simulink model "TRAS_PID_Cross"  (R2016a)
settings: Solver=ode5  SolverMode=SingleTasking  StartTime=0.0  StopTime=90  FixedStep=0.01  RelTol=1e-3  AbsTol=1e-6
settings Model: SimulationMode=external  ExtModeTrigDuration=12000  ExtModeTrigLevel=0.400000  Creator=jims  LastModifiedBy=inteco
settings DataIOCC: ExternalInput=[]  InitialState=[]  MaxDataPoints=5000  SaveFormat=Array  SignalLoggingSaveFormat=ModelDataLogs  SaveOutput=off  SaveTime=off  SignalLoggingName=sigsOut
settings OptimizationCC: BooleanDataType=off  ExpressionDepthLimit=2147483647  InitFltsAndDblsToZero=on
settings DebuggingCC: SaveWithParameterizedLinksMsg=none  UnderspecifiedInitializationDetection=Classic  MergeDetectMultiDrivingBlocksExec=none  SignalResolutionControl=TryResolveAllWithWarning  MultiTaskDSMMsg=warning  MultiTaskCondExecSysMsg=none  IntegerOverflowMsg=none  FcnCallInpInsideContextMsg=UseLocalSettings  StateNameClashWarn=warning  IntegerSaturationMsg=none
settings HardwareCC: ProdBitPerPointer=32  ProdLargestAtomicFloat=None  ProdIntDivRoundTo=Undefined  ProdEndianess=Unspecified  ProdWordSize=32  ProdHWDeviceType=32-bit Generic
settings ModelReferenceCC: PropagateSignalLabelsOutOfModel=off
settings RTWCC: SystemTargetFile=rtcon_tras_usb2.tlc  TemplateMakefile=rtcon_tras_vc_usb2_x64.tmf  Description=TRAS RTDAC/USB2 (Visual C/C++)
settings STFCustomTargetCC: ModelReferenceCompliant=off  GeneratePreprocessorConditionals=Disable all  CombineOutputUpdateFcns=on  MatFileLogging=on  CPPClassGenCompliant=on  GRTInterface=off  SystemTargetFile=rtcon_tras_usb2.tlc
settings GRTTargetCC: ModelReferenceCompliant=off  ParMdlRefBuildCompliant=off  CompOptLevelCompliant=off  ConcurrentExecutionCompliant=off  UseToolchainInfoCompliant=off  ExtMode=on  ExtModeMexFile=rtcon_ext_comm
settings ConfigComp: CovModelRefEnable=Off  CovSFcnEnable=off

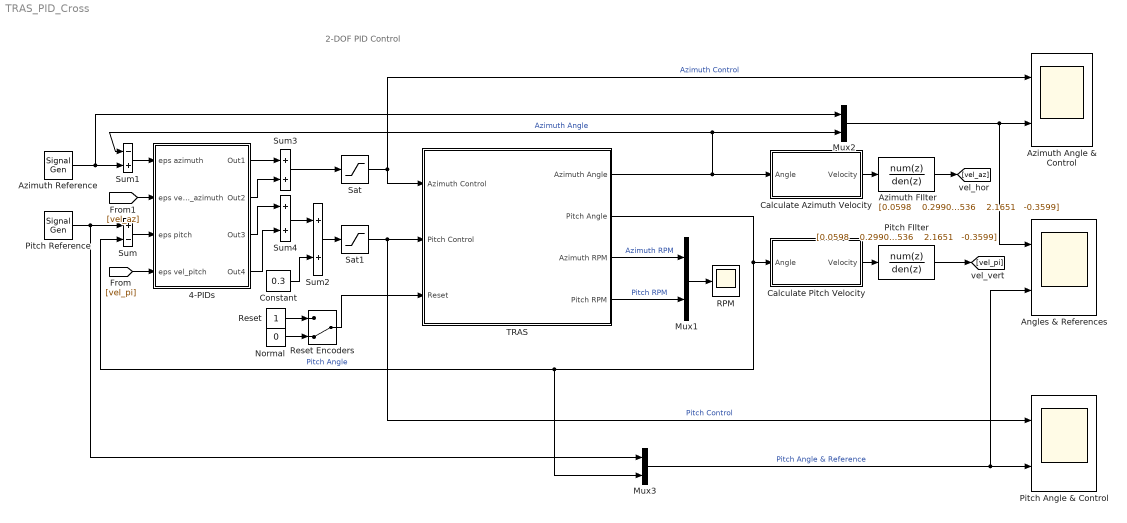
== system TRAS_PID_Cross ==
  note: 2-DOF PID Control
  4-PIDs : Subsystem  mask(4 PID controllers){phh=[1.9758/1.5 0.115 1.4008], pvh=[0 0 0.3], phv=[0 0 0.223], pvv=[0.0339 0.3532 0.7918]}
      mask prompts: phh "[Kphh Kihh Kdhh]"; pvh "[Kpvh Kivh Kdvh]"; phv "[Kphv Kihv Kdhv]"; pvv "[Kpvv Kivv Kdvv]"
      mask help: Parameters for cross-coupled PID controllers
      mask init:
      | Kphh = phh(1); Kihh = phh(2); Kdhh = phh(3);
      | Kpvh = pvh(1); Kivh = pvh(2); Kdvh = pvh(3);
      | Kphv = phv(1); Kihv = phv(2); Kdhv = phv(3);
      | Kpvv = pvv(1); Kivv = pvv(2); Kdvv = pvv(3);
      mask Help: Parameters for cross-coupled PID controllers
  Angles & References : Scope  NumInputPorts=2
  Azimuth Angle & Control : Scope  NumInputPorts=2
  Azimuth Reference : SignalGenerator  WaveForm=square  Amplitude=.4  Frequency=.02
  Azimuth FIlter : DiscreteTransferFcn  Numerator="[0.0598    0.2990    0.5980    0.5980    0.2990    0.0598] * 1e-3"  Denominator="[1.0000   -3.9845    6.4349   -5.2536    2.1651   -0.3599]"  SampleTime=0.01
  Calculate Azimuth Velocity : Subsystem
      mask Display: disp( 'rad-to-rad/s' )
  Calculate Pitch Velocity : Subsystem
      mask Display: disp( 'rad-to-rad/s' )
  Constant : Constant  Value=0.3
  Mux1 : Mux  Inputs=2
  Mux2 : Mux  Inputs=2
  Mux3 : Mux  Inputs=2
  Normal : Constant  Value=0
  Pitch Angle & Control : Scope  NumInputPorts=2
  Pitch Reference : SignalGenerator  Amplitude=.25  Frequency=1/60
  Pitch FIlter : DiscreteTransferFcn  Numerator="[0.0598    0.2990    0.5980    0.5980    0.2990    0.0598] * 1e-3"  Denominator="[1.0000   -3.9845    6.4349   -5.2536    2.1651   -0.3599]"  SampleTime=0.01
  RPM : Scope
  Reset : Constant
  Reset Encoders : ManualSwitch  CurrentSetting=0
  Sat : Saturate
  Sat1 : Saturate  UpperLimit=1  LowerLimit=0
  Sum : Sum  Inputs=+-  SaturateOnIntegerOverflow=on
  Sum1 : Sum  Inputs=-+  SaturateOnIntegerOverflow=on
  Sum2 : Sum  SaturateOnIntegerOverflow=on
  Sum3 : Sum  SaturateOnIntegerOverflow=on
  Sum4 : Sum  SaturateOnIntegerOverflow=on
  TRAS : Subsystem
      mask Display: image(imread('Tras.JPG'))
  wires:
  TRAS/1(Azimuth Angle) -> Mux2/2, Sum1/1, Calculate Azimuth Velocity/1(Angle)  "Azimuth Angle"
  TRAS/4(Pitch RPM) -> Mux1/2  "Pitch RPM"
  Normal/1 -> Reset Encoders/2
  Reset/1 -> Reset Encoders/1
  Reset Encoders/1 -> TRAS/3(Reset)
  Mux2/1 -> Angles & References/1, Azimuth Angle & Control/2
  Sum2/1 -> Sat1/1
  Sat1/1 -> Pitch Angle & Control/1, TRAS/2(Pitch Control)  "Pitch Control"
  Azimuth Reference/1 -> Sum1/2, Mux2/1
  Pitch Reference/1 -> Sum/1, Mux3/1
  Sat/1 -> Azimuth Angle & Control/1, TRAS/1(Azimuth Control)  "Azimuth Control"
  Constant/1 -> Sum2/2
  Sum3/1 -> Sat/1
  Sum4/1 -> Sum2/1
  Mux1/1 -> RPM/1
  TRAS/2(Pitch Angle) -> Sum/2, Mux3/2, Calculate Pitch Velocity/1(Angle)  "Pitch Angle"
  Mux3/1 -> Angles & References/2, Pitch Angle & Control/2  "Pitch Angle & Reference"
  Calculate Azimuth Velocity/1(Velocity) -> Azimuth FIlter/1
  Calculate Pitch Velocity/1(Velocity) -> Pitch FIlter/1
  Sum1/1 -> 4-PIDs/1(eps azimuth)
  Sum/1 -> 4-PIDs/3(eps pitch)
  Azimuth FIlter/1 -> [vel_az]
  Pitch FIlter/1 -> [vel_pi]
  4-PIDs/1(Out1) -> Sum3/1
  4-PIDs/2(Out2) -> Sum3/2
  4-PIDs/3(Out3) -> Sum4/1
  4-PIDs/4(Out4) -> Sum4/2
  [vel_az] -> 4-PIDs/2(eps vel_azimuth)
  [vel_pi] -> 4-PIDs/4(eps vel_pitch)
  TRAS/3(Azimuth RPM) -> Mux1/1  "Azimuth RPM"

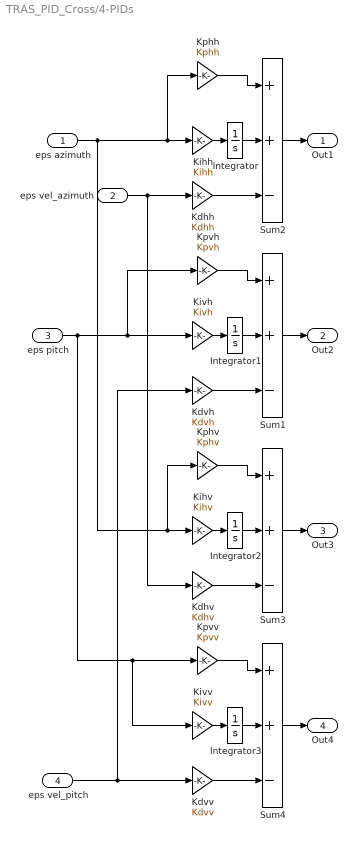
== system TRAS_PID_Cross/4-PIDs ==
  eps azimuth : Inport
  eps vel_azimuth : Inport  Port=2
  eps pitch : Inport  Port=3
  eps vel_pitch : Inport  Port=4
  Integrator : Integrator  LimitOutput=on  UpperSaturationLimit=0.5  LowerSaturationLimit=-0.5
  Integrator1 : Integrator  LimitOutput=on
  Integrator2 : Integrator
  Integrator3 : Integrator  LimitOutput=on  UpperSaturationLimit=0.25  LowerSaturationLimit=-0.25
  Kdhh : Gain  Gain=Kdhh  SaturateOnIntegerOverflow=on  OutDataTypeStr=Inherit: Same as input  ParamDataTypeStr=Inherit: Same as input
  Kdhv : Gain  Gain=Kdhv  SaturateOnIntegerOverflow=on  OutDataTypeStr=Inherit: Same as input  ParamDataTypeStr=Inherit: Same as input
  Kdvh : Gain  Gain=Kdvh  SaturateOnIntegerOverflow=on  OutDataTypeStr=Inherit: Same as input  ParamDataTypeStr=Inherit: Same as input
  Kdvv : Gain  Gain=Kdvv  SaturateOnIntegerOverflow=on  OutDataTypeStr=Inherit: Same as input  ParamDataTypeStr=Inherit: Same as input
  Kihh : Gain  Gain=Kihh  SaturateOnIntegerOverflow=on  OutDataTypeStr=Inherit: Same as input  ParamDataTypeStr=Inherit: Same as input
  Kihv : Gain  Gain=Kihv  SaturateOnIntegerOverflow=on  OutDataTypeStr=Inherit: Same as input  ParamDataTypeStr=Inherit: Same as input
  Kivh : Gain  Gain=Kivh  SaturateOnIntegerOverflow=on  OutDataTypeStr=Inherit: Same as input  ParamDataTypeStr=Inherit: Same as input
  Kivv : Gain  Gain=Kivv  SaturateOnIntegerOverflow=on  OutDataTypeStr=Inherit: Same as input  ParamDataTypeStr=Inherit: Same as input
  Kphh : Gain  Gain=Kphh  SaturateOnIntegerOverflow=on  OutDataTypeStr=Inherit: Same as input  ParamDataTypeStr=Inherit: Same as input
  Kphv : Gain  Gain=Kphv  SaturateOnIntegerOverflow=on  OutDataTypeStr=Inherit: Same as input  ParamDataTypeStr=Inherit: Same as input
  Kpvh : Gain  Gain=Kpvh  SaturateOnIntegerOverflow=on  OutDataTypeStr=Inherit: Same as input  ParamDataTypeStr=Inherit: Same as input
  Kpvv : Gain  Gain=Kpvv  SaturateOnIntegerOverflow=on  OutDataTypeStr=Inherit: Same as input  ParamDataTypeStr=Inherit: Same as input
  Sum{1..4} (4 alike) : Sum  Inputs=++-  SaturateOnIntegerOverflow=on  InputSameDT=on  OutDataTypeStr=Inherit: Same as first input
  Out1 : Outport
  Out2 : Outport  Port=2
  Out3 : Outport  Port=3
  Out4 : Outport  Port=4
  wires:
  Sum4/1 -> Out4/1
  Sum3/1 -> Out3/1
  Sum1/1 -> Out2/1
  Sum2/1 -> Out1/1
  Kdvv/1 -> Sum4/3
  Kivv/1 -> Integrator3/1
  Integrator3/1 -> Sum4/2
  Kpvv/1 -> Sum4/1
  Kdhv/1 -> Sum3/3
  Kihv/1 -> Integrator2/1
  Integrator2/1 -> Sum3/2
  Kphv/1 -> Sum3/1
  Kdvh/1 -> Sum1/3
  Kivh/1 -> Integrator1/1
  Integrator1/1 -> Sum1/2
  Kpvh/1 -> Sum1/1
  Kdhh/1 -> Sum2/3
  Kihh/1 -> Integrator/1
  Integrator/1 -> Sum2/2
  Kphh/1 -> Sum2/1
  eps azimuth/1 -> Kihv/1, Kphv/1, Kihh/1, Kphh/1
  eps vel_azimuth/1 -> Kdhv/1, Kdhh/1
  eps pitch/1 -> Kivh/1, Kpvh/1, Kpvv/1, Kivv/1
  eps vel_pitch/1 -> Kdvv/1, Kdvh/1

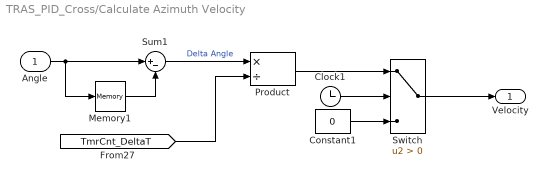
== system TRAS_PID_Cross/Calculate Azimuth Velocity ==
  Angle : Inport
  Clock1 : Clock
  Constant1 : Constant  Value=0
  Memory1 : Memory
  Product : Product  Inputs=*/  SaturateOnIntegerOverflow=on  InputSameDT=on  OutDataTypeStr=Inherit: Same as first input
  Sum1 : Sum  Inputs=|+-  SaturateOnIntegerOverflow=on  InputSameDT=on  OutDataTypeStr=Inherit: Same as first input
  Switch : Switch  Criteria=u2 > Threshold  SaturateOnIntegerOverflow=on  InputSameDT=on
  Velocity : Outport
  wires:
  [TmrCnt_DeltaT] -> Product/2
  Memory1/1 -> Sum1/2
  Angle/1 -> Sum1/1, Memory1/1
  Sum1/1 -> Product/1  "Delta Angle"
  Product/1 -> Switch/1
  Clock1/1 -> Switch/2
  Constant1/1 -> Switch/3
  Switch/1 -> Velocity/1

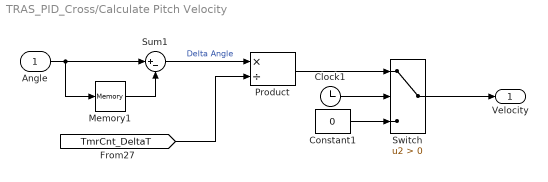
== system TRAS_PID_Cross/Calculate Pitch Velocity ==
  Angle : Inport
  Clock1 : Clock
  Constant1 : Constant  Value=0
  Memory1 : Memory
  Product : Product  Inputs=*/  SaturateOnIntegerOverflow=on  InputSameDT=on  OutDataTypeStr=Inherit: Same as first input
  Sum1 : Sum  Inputs=|+-  SaturateOnIntegerOverflow=on  InputSameDT=on  OutDataTypeStr=Inherit: Same as first input
  Switch : Switch  Criteria=u2 > Threshold  SaturateOnIntegerOverflow=on  InputSameDT=on
  Velocity : Outport
  wires:
  Switch/1 -> Velocity/1
  Constant1/1 -> Switch/3
  Clock1/1 -> Switch/2
  Product/1 -> Switch/1
  Sum1/1 -> Product/1  "Delta Angle"
  Angle/1 -> Memory1/1, Sum1/1
  Memory1/1 -> Sum1/2
  [TmrCnt_DeltaT] -> Product/2

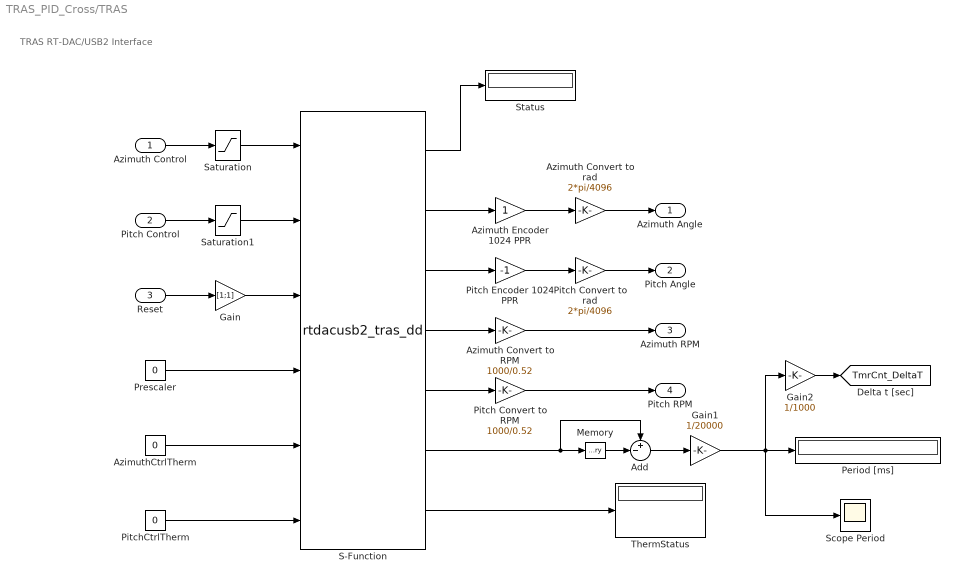
== system TRAS_PID_Cross/TRAS ==
  note: TRAS RT-DAC/USB2
      | Interface
  Azimuth Control : Inport
  Pitch Control : Inport  Port=2
  Reset : Inport  Port=3
  Add : Sum  Inputs=+-|
  Azimuth Convert to RPM : Gain  Gain=1000/0.52  SaturateOnIntegerOverflow=on  OutDataTypeStr=Inherit: Same as input  ParamDataTypeStr=Inherit: Same as input
  Azimuth Convert to rad : Gain  Gain=2*pi/4096  SaturateOnIntegerOverflow=on  OutDataTypeStr=Inherit: Same as input  ParamDataTypeStr=Inherit: Same as input
  Azimuth Encoder 1024 PPR : Gain  SaturateOnIntegerOverflow=on  OutDataTypeStr=Inherit: Same as input  ParamDataTypeStr=Inherit: Same as input
  AzimuthCtrlTherm : Constant  Value=0
  Gain : Gain  Gain=[1;1]
  Gain1 : Gain  Gain=1/20000
  Gain2 : Gain  Gain=1/1000
  Memory : Memory
  Period [ms] : Display
  Pitch Convert to RPM : Gain  Gain=1000/0.52  SaturateOnIntegerOverflow=on  OutDataTypeStr=Inherit: Same as input  ParamDataTypeStr=Inherit: Same as input
  Pitch Convert to rad : Gain  Gain=2*pi/4096  SaturateOnIntegerOverflow=on  OutDataTypeStr=Inherit: Same as input  ParamDataTypeStr=Inherit: Same as input
  Pitch Encoder 1024 PPR : Gain  Gain=-1  SaturateOnIntegerOverflow=on  OutDataTypeStr=Inherit: Same as input  ParamDataTypeStr=Inherit: Same as input
  PitchCtrlTherm : Constant  Value=0
  Prescaler : Constant  Value=0
  S-Function : S-Function  FunctionName=rtdacusb2_tras_dd  Parameters=1, 0.01  SFunctionDeploymentMode=off  EnableBusSupport=off
  Saturation : Saturate  UpperLimit=1  LowerLimit=-1
  Saturation1 : Saturate  UpperLimit=1  LowerLimit=-1
  Scope Period : Scope
  Status : Display
  ThermStatus : Display
  Azimuth Angle : Outport
  Pitch Angle : Outport  Port=2
  Azimuth RPM : Outport  Port=3
  Pitch RPM : Outport  Port=4
  tag scope: TmrCnt_DeltaT=global
  wires:
  Gain2/1 -> [TmrCnt_DeltaT]
  Gain1/1 -> Gain2/1, Period [ms]/1, Scope Period/1
  S-Function/6 -> Add/1, Memory/1
  Add/1 -> Gain1/1
  Memory/1 -> Add/2
  S-Function/7 -> ThermStatus/1
  Pitch Convert to RPM/1 -> Pitch RPM/1
  Azimuth Convert to RPM/1 -> Azimuth RPM/1
  S-Function/5 -> Pitch Convert to RPM/1
  S-Function/4 -> Azimuth Convert to RPM/1
  Pitch Convert to rad/1 -> Pitch Angle/1
  S-Function/3 -> Pitch Encoder 1024 PPR/1
  Pitch Encoder 1024 PPR/1 -> Pitch Convert to rad/1
  Azimuth Convert to rad/1 -> Azimuth Angle/1
  S-Function/2 -> Azimuth Encoder 1024 PPR/1
  Azimuth Encoder 1024 PPR/1 -> Azimuth Convert to rad/1
  S-Function/1 -> Status/1
  Gain/1 -> S-Function/3
  Saturation1/1 -> S-Function/2
  Saturation/1 -> S-Function/1
  PitchCtrlTherm/1 -> S-Function/6
  AzimuthCtrlTherm/1 -> S-Function/5
  Prescaler/1 -> S-Function/4
  Reset/1 -> Gain/1
  Pitch Control/1 -> Saturation1/1
  Azimuth Control/1 -> Saturation/1
